simulink model "AdaptiveRobust"  (R2022b)
settings: Solver=VariableStepAuto  StartTime=0.0  StopTime=50  RelTol=1e-3
undefined symbols (not defined in the file): A_sys, Am, b_sys, bm, cm, k, lambda, P, sigma, Theta
settings Model: Creator=zein  LastModifiedBy=zein

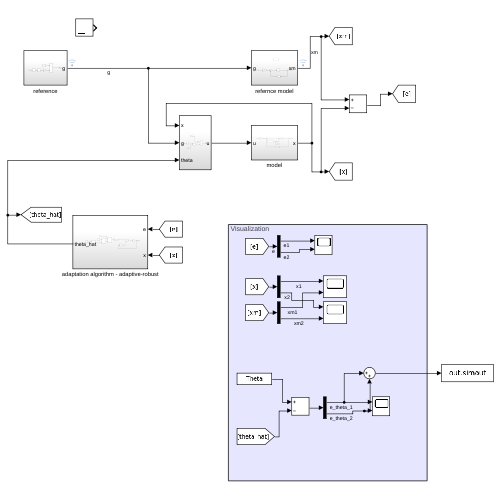
[thumbnail: Simulink's stored preview of the top-level diagram]
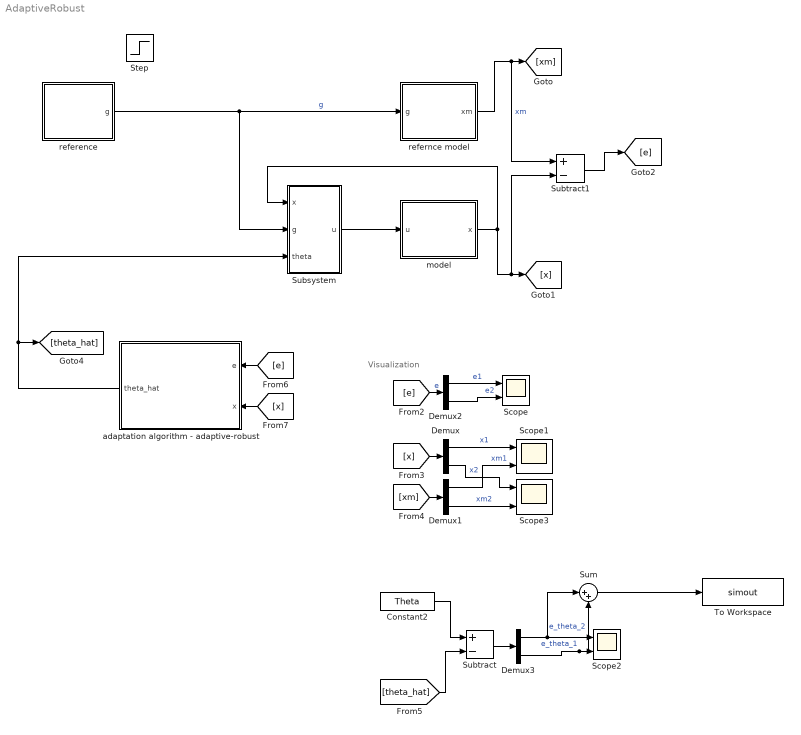
== system AdaptiveRobust ==
  note: Visualization
  Constant2 : Constant  Value=Theta
  Demux{,1..3} (4 alike) : Demux  Outputs=2
  Scope{,1..3} (4 alike) : Scope  NumInputPorts=2
  Step : Step  Time=0  SampleTime=0
  Subsystem : Subsystem
  Subtract : Sum  Inputs=+-
  Subtract1 : Sum  Inputs=+-
  Sum : Sum  Inputs=|++
  To Workspace : ToWorkspace  VariableName=simout  SaveFormat=Timeseries  SampleTime=-1
  adaptation algorithm - adaptive-robust : Subsystem
  model : Subsystem
  reference : Subsystem
  refernce model : Subsystem
  wires:
  reference/1(g) -> Subsystem/2(g), refernce model/1(g)  "g"
  refernce model/1(xm) -> Subtract1/1, [xm]  "xm"
  Subsystem/1(u) -> model/1(u)
  Subtract1/1 -> [e]
  [e] -> Demux2/1  "e"
  Constant2/1 -> Subtract/1
  [theta_hat] -> Subtract/2
  Subtract/1 -> Demux3/1
  [x] -> Demux/1
  [xm] -> Demux1/1
  Demux/1 -> Scope1/1  "x1"
  Demux/2 -> Scope3/1  "x2"
  Demux1/1 -> Scope1/2  "xm1"
  Demux1/2 -> Scope3/2  "xm2"
  model/1(x) -> Subsystem/1(x), Subtract1/2, [x]
  Demux2/1 -> Scope/1  "e1"
  Demux2/2 -> Scope/2  "e2"
  Demux3/1 -> Sum/1, Scope2/1  "e_theta_1"
  Demux3/2 -> Sum/2, Scope2/2  "e_theta_2"
  Sum/1 -> To Workspace/1
  adaptation algorithm - adaptive-robust/1(theta_hat) -> Subsystem/3(theta), [theta_hat]
  [e] -> adaptation algorithm - adaptive-robust/1(e)
  [x] -> adaptation algorithm - adaptive-robust/2(x)

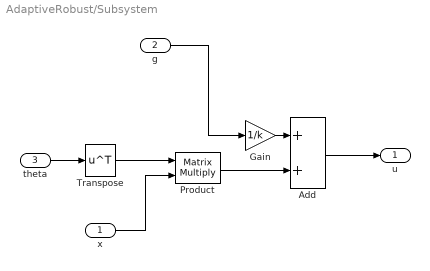
== system AdaptiveRobust/Subsystem ==
  x : Inport
  g : Inport  Port=2
  theta : Inport  Port=3
  Add : Sum
  Gain : Gain  Gain=1/k
  Product : Product  Multiplication=Matrix(*)
  Transpose : Math  Operator=transpose
  u : Outport
  wires:
  g/1 -> Gain/1
  Product/1 -> Add/2
  x/1 -> Product/2
  Add/1 -> u/1
  Gain/1 -> Add/1
  theta/1 -> Transpose/1
  Transpose/1 -> Product/1

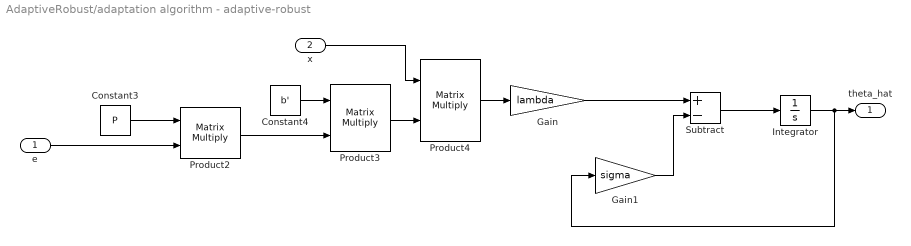
== system AdaptiveRobust/adaptation algorithm - adaptive-robust ==
  e : Inport
  x : Inport  Port=2
  Constant3 : Constant  Value=P  VectorParams1D=off
  Constant4 : Constant  Value=b'  VectorParams1D=off
  Gain : Gain  Gain=lambda
  Gain1 : Gain  Gain=sigma
  Integrator : Integrator
  Product2 : Product  Multiplication=Matrix(*)
  Product3 : Product  Multiplication=Matrix(*)
  Product4 : Product  Multiplication=Matrix(*)
  Subtract : Sum  Inputs=+-
  theta_hat : Outport
  wires:
  Product2/1 -> Product3/2
  Product3/1 -> Product4/2
  Product4/1 -> Gain/1
  Constant4/1 -> Product3/1
  e/1 -> Product2/2
  Gain/1 -> Subtract/1
  Constant3/1 -> Product2/1
  x/1 -> Product4/1
  Integrator/1 -> Gain1/1, theta_hat/1
  Subtract/1 -> Integrator/1
  Gain1/1 -> Subtract/2

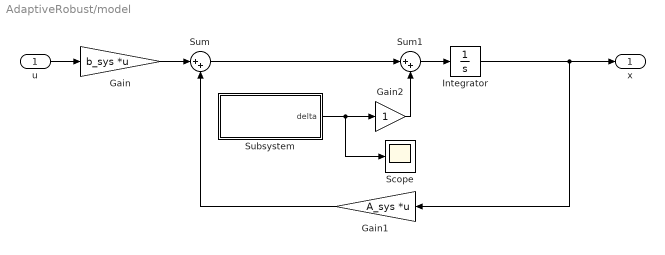
== system AdaptiveRobust/model ==
  u : Inport
  Gain : Gain  Gain=b_sys  Multiplication=Matrix(K*u)
  Gain1 : Gain  Gain=A_sys  Multiplication=Matrix(K*u)
  Gain2 : Gain
  Integrator : Integrator  InitialCondition=[0;0]
  Scope : Scope
  Subsystem : Subsystem
  Sum : Sum  Inputs=|++
  Sum1 : Sum  Inputs=|++
  x : Outport
  wires:
  u/1 -> Gain/1
  Integrator/1 -> x/1, Gain1/1
  Sum/1 -> Sum1/1
  Gain1/1 -> Sum/2
  Gain/1 -> Sum/1
  Sum1/1 -> Integrator/1
  Subsystem/1(delta) -> Scope/1, Gain2/1
  Gain2/1 -> Sum1/2

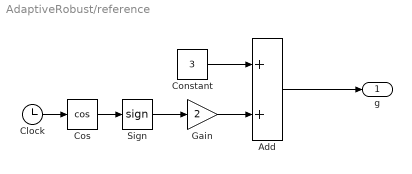
== system AdaptiveRobust/reference ==
  Add : Sum
  Clock : Clock
  Constant : Constant  Value=3
  Cos : Trigonometry  Operator=cos
  Gain : Gain  Gain=2
  Sign : Signum
  g : Outport
  wires:
  Clock/1 -> Cos/1
  Sign/1 -> Gain/1
  Constant/1 -> Add/1
  Add/1 -> g/1
  Cos/1 -> Sign/1
  Gain/1 -> Add/2

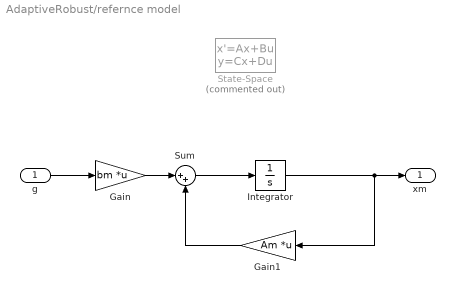
== system AdaptiveRobust/refernce model ==
  g : Inport
  Gain : Gain  Gain=bm  Multiplication=Matrix(K*u)
  Gain1 : Gain  Gain=Am  Multiplication=Matrix(K*u)
  Integrator : Integrator  InitialCondition=[0;0]
  State-Space : StateSpace  Commented=on  A=Am  B=bm  C=cm  D=0  InitialCondition=0
  Sum : Sum  Inputs=|++
  xm : Outport
  wires:
  Integrator/1 -> Gain1/1, xm/1
  g/1 -> Gain/1
  Gain/1 -> Sum/1
  Gain1/1 -> Sum/2
  Sum/1 -> Integrator/1

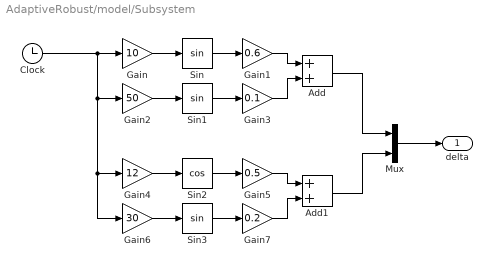
== system AdaptiveRobust/model/Subsystem ==
  Add : Sum
  Add1 : Sum
  Clock : Clock
  Gain : Gain  Gain=10
  Gain1 : Gain  Gain=0.6
  Gain2 : Gain  Gain=50
  Gain3 : Gain  Gain=0.1
  Gain4 : Gain  Gain=12
  Gain5 : Gain  Gain=0.5
  Gain6 : Gain  Gain=30
  Gain7 : Gain  Gain=0.2
  Mux : Mux  Inputs=2
  Sin : Trigonometry
  Sin1 : Trigonometry
  Sin2 : Trigonometry  Operator=cos
  Sin3 : Trigonometry
  delta : Outport
  wires:
  Gain/1 -> Sin/1
  Sin/1 -> Gain1/1
  Sin1/1 -> Gain3/1
  Gain2/1 -> Sin1/1
  Gain1/1 -> Add/1
  Gain3/1 -> Add/2
  Gain7/1 -> Add1/2
  Gain5/1 -> Add1/1
  Gain6/1 -> Sin3/1
  Sin3/1 -> Gain7/1
  Sin2/1 -> Gain5/1
  Gain4/1 -> Sin2/1
  Clock/1 -> Gain4/1, Gain6/1, Gain2/1, Gain/1
  Add/1 -> Mux/1
  Add1/1 -> Mux/2
  Mux/1 -> delta/1
